simulink model "model_ej3"  (R2023b)
settings: Solver=FixedStepAuto  StartTime=0.0  StopTime=2  FixedStep=step  RelTol=1e-3
values from neighbouring files (symbols this model uses):
  Kp = 100    [EJ3.m]
  Kv = 2000    [EJ3.m]
  robot = SerialLink(L, 'tool', Tool)    [EJ3.m]
undefined symbols (not defined in the file or in its folder): gravload, inertia, qc
libraries: roblocks x8
settings Model: Creator=ohvic  LastModifiedBy=alero
settings DebuggingCC: UnconnectedInputMsg=warning  UnconnectedOutputMsg=warning  UnconnectedLineMsg=warning
settings ModelReferenceCC: EnableRefExpFcnMdlSchedulingChecks=on
settings RTWCC: DLArmComputeVersion=19.05

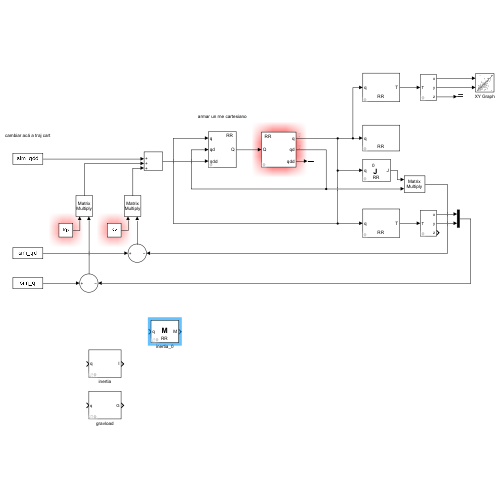
[thumbnail: Simulink's stored preview of the top-level diagram]
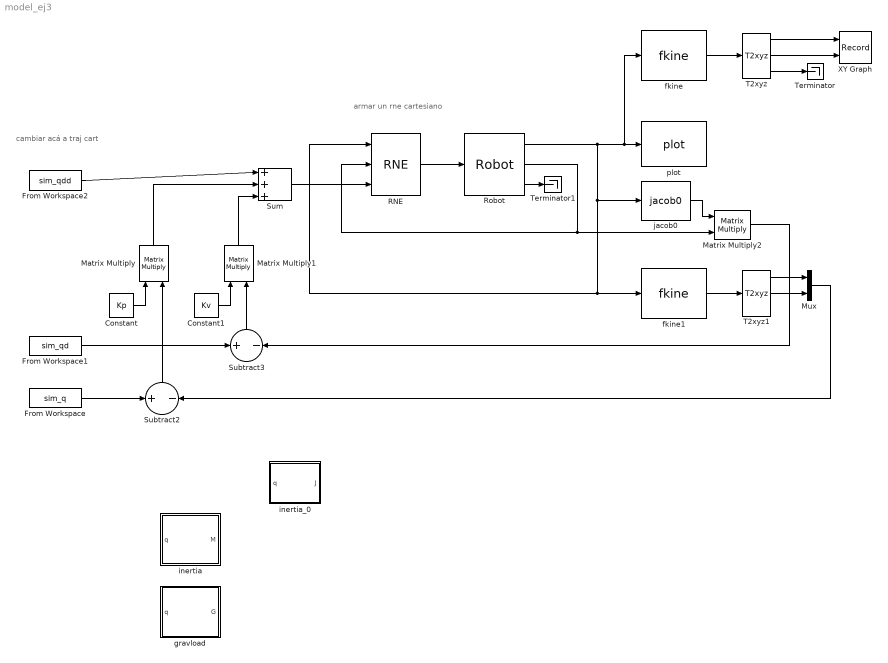
== system model_ej3 ==
  note: armar un rne cartesiano
  note: cambiar acá a traj cart
  Constant : Constant  Value=Kp
  Constant1 : Constant  Value=Kv
  From Workspace : FromWorkspace  VariableName=sim_q  SampleTime=step
  From Workspace1 : FromWorkspace  VariableName=sim_qd  SampleTime=step
  From Workspace2 : FromWorkspace  VariableName=sim_qdd  SampleTime=step
  Matrix Multiply : Product  Multiplication=Matrix(*)
  Matrix Multiply1 : Product  Multiplication=Matrix(*)
  Matrix Multiply2 : Product  Multiplication=Matrix(*)
  Mux : Mux  Inputs=2
  RNE : roblocks/Arm/RNE  robot=robot  grav=[0 0 9.81]
  Robot : roblocks/Arm/Robot  robot=robot  q0=qc(1,:)
  Subtract2 : Sum  Inputs=+-
  Subtract3 : Sum  Inputs=+-
  Sum : Sum  Inputs=|+++
  T2xyz : roblocks/Toolbox/T2xyz
  T2xyz1 : roblocks/Toolbox/T2xyz
  Terminator : Terminator
  Terminator1 : Terminator
  XY Graph : Record  FileSettingsInternal="{\"entries\":[{\"content\":{\"excelSettings\":{\"content\":{},\"type\":\"Streamout.ExcelSettings\"}},\"type\":\"Streamout.FileSettingStorage\",\"uuid\":\"\"}],\"packageUris\":[\"http:\\/\\/schema.mathworks.com\\/mf0\\/streamout_blocks\\/R2020a\"],\"version\":\"1.0\"}"  Layout=[1 1]  SignalsInternal="{\"entries\":[{\"content\":{\"signals\":[{\"content\":{\"blockPath\":[],\"dimensions\":[1],\"domain\":\"\",\"lineColor\":\"#a2142f\",\"plots\":[1],\"port\":1,\"signalID\":20,\"signalName\":\"XY Graph:1\"},\"type\":\"RecordBlkView.Signal\",\"uuid\":\"\"},{\"content\":{\"blockPath\":[],\"dimensions\":[1],\"domain\":\"\",\"lineColor\":\"#139fff\",\"plots\":[1],\"port\":2,\"signalID\":23,\"signalName\":\"XY Graph:2\"},\"type\":\"RecordBlkView.Signal\",\"uuid\":\"\"}]},\"type\":\"RecordBlkView.InputSignals\",\"uuid\":\"\"}],\"packageUris\":[\"http:\\/\\/schema.mathworks.com\\/mf0\\/streamout_blocks\\/R2020a\"],\"version\":\"1.0\"}"  VisualizationBindings="{\"xyplotplugin\":{\"info\":[{\"series\":[{\"bindingParametersList\":[{\"parameter\":\"X-Axis\",\"signalID\":20,\"signalName\":\"XY Graph:1\"},{\"parameter\":\"Y-Axis\",\"signalID\":23,\"signalName\":\"XY Graph:2\"}],\"seriesID\":32213}],\"subplotID\":1}]}}"  CompatibilityTag=XY  st=-1
  fkine : roblocks/Arm/fkine  robot=robot
  fkine1 : roblocks/Arm/fkine  robot=robot
  gravload : Subsystem  AncestorBlock=roblocks/Arm/gravload  mask{robot=robot}
  inertia : Subsystem  AncestorBlock=roblocks/Arm/inertia  mask{robot=robot}
      mask Display:
      | text(0.5, 0.2, '\bf\fontsize{16}M', 'texmode', 'on', 'verticalAlignment', 'middle', 'horizontalAlignment', 'center')
      | %text(0.45, 0.65, '\fontsize{10}0', 'texmode', 'on','verticalAlignment', 'bottom', 'horizontalAlignment', 'right')
      | if ~isempty(robot)
      |     text(0.5, 0.2, robot.name,  'horizontalAlignment', 'center')
      | end
      | port_label('input', 1, 'q')
      | port_label('output', 1, 'I')
  inertia_0 : Subsystem  AncestorBlock=roblocks/Arm/jacob0  mask{robot=robot}
      mask prompts: robot "Robot object"
      mask help: Robot Jacobian in world coordinates
      mask init:
      | if ~isempty(robot)
      |     n=robot.n;
      | end
      mask Help:
      | Jacobian matrix relating joint coordinate rates to end-effector spatial
      | velocity expressed in the world frame.
      | 
      | <b>Parameters::</b>
      | 
      | Robot (SerialLink class)  The N-axis robot object for which the Jacobian is
      |                           computed.
      | 
      | <b>Inputs::</b>
      | 
      | q (1xN) joint coordinates
      | 
      | <b>Outputs::</b>
      | 
      | J (6xN) the Jacobian matrix
      | 
      | <b>Notes::</b>
      | 
      | - A wrapper for the Toolbox method jacob0().
      mask Display:
      | text(0.4, 0.8, '\bf\fontsize{16}M', 'texmode', 'on', 'verticalAlignment', 'top', 'horizontalAlignment', 'left')
      | %text(0.45, 0.65, '\fontsize{10}0', 'texmode', 'on','verticalAlignment', 'bottom', 'horizontalAlignment', 'right')
      | if ~isempty(robot)
      |     text(0.5, 0.2, robot.name,  'horizontalAlignment', 'center')
      | end
      | port_label('input', 1, 'q')
      | port_label('output', 1, 'M')
  "jacob0 " : roblocks/Arm/jacob0   robot=robot
  plot : roblocks/Arm/plot  robot=robot  fps=25  holdplot=off
  wires:
  Constant/1 -> Matrix Multiply/1
  Constant1/1 -> Matrix Multiply1/1
  From Workspace/1 -> Subtract2/1
  From Workspace1/1 -> Subtract3/1
  Subtract2/1 -> Matrix Multiply/2
  Subtract3/1 -> Matrix Multiply1/2
  From Workspace2/1 -> Sum/1
  Matrix Multiply/1 -> Sum/2
  Matrix Multiply1/1 -> Sum/3
  Robot/3 -> Terminator1/1
  T2xyz/1 -> XY Graph/1
  T2xyz/2 -> XY Graph/2
  fkine/1 -> T2xyz/1
  T2xyz/3 -> Terminator/1
  Robot/2 -> RNE/2, Matrix Multiply2/2
  Robot/1 -> fkine/1, plot/1, RNE/1, fkine1/1, "jacob0 "/1
  Sum/1 -> RNE/3
  RNE/1 -> Robot/1
  "jacob0 "/1 -> Matrix Multiply2/1
  fkine1/1 -> T2xyz1/1
  T2xyz1/1 -> Mux/1
  T2xyz1/2 -> Mux/2
  Mux/1 -> Subtract2/2
  Matrix Multiply2/1 -> Subtract3/2

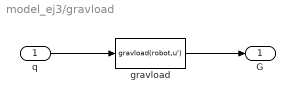
== system model_ej3/gravload ==
  q : Inport
  gravload : MATLABFcn  MATLABFcn=gravload(robot,u')  OutputDimensions=[1 robot.n]  Output1D=off
  G : Outport  VectorParamsAs1DForOutWhenUnconnected=off
  wires:
  q/1 -> gravload/1
  gravload/1 -> G/1

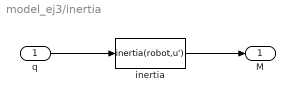
== system model_ej3/inertia ==
  q : Inport
  inertia : MATLABFcn  MATLABFcn=inertia(robot,u')  OutputDimensions=[robot.n robot.n]  Output1D=off
  M : Outport  VectorParamsAs1DForOutWhenUnconnected=off
  wires:
  q/1 -> inertia/1
  inertia/1 -> M/1

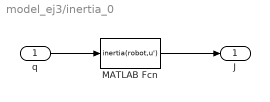
== system model_ej3/inertia_0 ==
  q : Inport
  MATLAB Fcn : MATLABFcn  MATLABFcn=inertia(robot,u')  OutputDimensions=[robot.n robot.n]  Output1D=off
  J : Outport  VectorParamsAs1DForOutWhenUnconnected=off
  wires:
  MATLAB Fcn/1 -> J/1
  q/1 -> MATLAB Fcn/1
